simulink library "Multibody_Multiphysics_Lib"  (R2019a)
settings: Solver=ode45  StartTime=0.0  StopTime=10.0  RelTol=1e-3  EnableMultiTasking=on
undefined symbols (not defined in the file): pst_rOut, rod_rOut, stroke
libraries: fl_lib x51, forcesPS_lib x21, sm_lib x15, $bdroot x4
(part 2 of 2)

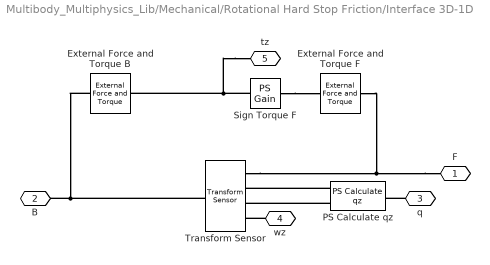
== system Multibody_Multiphysics_Lib/Mechanical/Rotational Hard Stop Friction/Interface 3D-1D ==
  External Force and Torque B : sm_lib/Forces and Torques/External Force and Torque  ForceResolutionFrame=AttachedFrame  EnableForceX=off  EnableForceY=off  EnableForceZ=off  EnableForce=off  TorqueResolutionFrame=AttachedFrame  EnableTorqueX=off  EnableTorqueY=off  EnableTorqueZ=on  EnableTorque=off
  External Force and Torque F : sm_lib/Forces and Torques/External Force and Torque  ForceResolutionFrame=AttachedFrame  EnableForceX=off  EnableForceY=off  EnableForceZ=off  EnableForce=off  TorqueResolutionFrame=AttachedFrame  EnableTorqueX=off  EnableTorqueY=off  EnableTorqueZ=on  EnableTorque=off
  PS Calculate qz : forcesPS_lib/Math/PS Calculate qz
  Sign Torque F : fl_lib/Physical Signals/Functions/PS Gain  gain=-1
  Transform Sensor : sm_lib/Frames and Transforms/Transform Sensor  MeasurementFrame=Base  SenseAngle=on  SenseAxis=on  SenseAngle1=off  SenseAngle2=off  SenseAngle3=off  SenseQ=off  SenseR=off  SenseOmegaX=off  SenseOmegaY=off  SenseOmegaZ=on  SenseOmega1=off  SenseOmega2=off  SenseOmega3=off  SenseQDot=off  SenseRDot=off  SenseAlphaX=off  SenseAlphaY=off  SenseAlphaZ=off  SenseAlpha1=off  SenseAlpha2=off  SenseAlpha3=off  SenseQDDot=off  SenseRDDot=off  SenseX=off  SenseY=off  SenseZ=off  SenseRad=off  SenseAzim=off  SenseDist=off  SenseInc=off  SenseXDot=off  SenseYDot=off  SenseZDot=off  SenseRadDot=off  SenseAzimDot=off  SenseDistDot=off  SenseIncDot=off  SenseXDDot=off  SenseYDDot=off  SenseZDDot=off  SenseRadDDot=off  SenseAzimDDot=off  SenseDistDDot=off  SenseIncDDot=off
  F : PMIOPort  Side=Right
  B : PMIOPort  Port=2  Side=Left
  q : PMIOPort  Port=3  Side=Left
  wz : PMIOPort  Port=4  Side=Left
  tz : PMIOPort  Port=5  Side=Right
  connections:
  q/RConn1 -- PS Calculate qz/RConn1
  PS Calculate qz/LConn2 -- Transform Sensor/RConn3
  PS Calculate qz/LConn1 -- Transform Sensor/RConn2
  tz/RConn1 -- External Force and Torque B/LConn1 -- Sign Torque F/LConn1
  Sign Torque F/RConn1 -- External Force and Torque F/LConn1
  wz/RConn1 -- Transform Sensor/RConn4
  External Force and Torque B/RConn1 -- B/RConn1 -- Transform Sensor/LConn1
  F/RConn1 -- Transform Sensor/RConn1 -- External Force and Torque F/RConn1

== system Multibody_Multiphysics_Lib/Mechanical/Translational Hard Stop Friction/Interface 3D-1D ==
  External Force and Torque B : sm_lib/Forces and Torques/External Force and Torque  ForceResolutionFrame=AttachedFrame  EnableForceX=off  EnableForceY=off  EnableForceZ=on  EnableForce=off  TorqueResolutionFrame=AttachedFrame  EnableTorqueX=off  EnableTorqueY=off  EnableTorqueZ=off  EnableTorque=off
  External Force and Torque F : sm_lib/Forces and Torques/External Force and Torque  ForceResolutionFrame=AttachedFrame  EnableForceX=off  EnableForceY=off  EnableForceZ=on  EnableForce=off  TorqueResolutionFrame=AttachedFrame  EnableTorqueX=off  EnableTorqueY=off  EnableTorqueZ=off  EnableTorque=off
  Sign Force F : fl_lib/Physical Signals/Functions/PS Gain  gain=-1
  Transform Sensor : sm_lib/Frames and Transforms/Transform Sensor  MeasurementFrame=Base  SenseAngle=off  SenseAxis=off  SenseAngle1=off  SenseAngle2=off  SenseAngle3=off  SenseQ=off  SenseR=off  SenseOmegaX=off  SenseOmegaY=off  SenseOmegaZ=off  SenseOmega1=off  SenseOmega2=off  SenseOmega3=off  SenseQDot=off  SenseRDot=off  SenseAlphaX=off  SenseAlphaY=off  SenseAlphaZ=off  SenseAlpha1=off  SenseAlpha2=off  SenseAlpha3=off  SenseQDDot=off  SenseRDDot=off  SenseX=off  SenseY=off  SenseZ=on  SenseRad=off  SenseAzim=off  SenseDist=off  SenseInc=off  SenseXDot=off  SenseYDot=off  SenseZDot=on  SenseRadDot=off  SenseAzimDot=off  SenseDistDot=off  SenseIncDot=off  SenseXDDot=off  SenseYDDot=off  SenseZDDot=off  SenseRadDDot=off  SenseAzimDDot=off  SenseDistDDot=off  SenseIncDDot=off
  F : PMIOPort  Side=Right
  B : PMIOPort  Port=2  Side=Left
  z : PMIOPort  Port=3  Side=Left
  vz : PMIOPort  Port=4  Side=Left
  fz : PMIOPort  Port=5  Side=Right
  connections:
  Transform Sensor/RConn1 -- F/RConn1 -- External Force and Torque F/RConn1
  Transform Sensor/LConn1 -- B/RConn1 -- External Force and Torque B/RConn1
  z/RConn1 -- Transform Sensor/RConn2
  vz/RConn1 -- Transform Sensor/RConn3
  Sign Force F/RConn1 -- External Force and Torque F/LConn1
  Sign Force F/LConn1 -- External Force and Torque B/LConn1 -- fz/RConn1
